simulink model "cordict1"  (R2023a)
settings: Solver=FixedStepAuto  StartTime=0.0  StopTime=60e-6  RelTol=1e-3
values from neighbouring files (symbols this model uses):
  FFTLength = 32    [matlab_channel.m]
  yr_c = yr_c(t,:)    [matlab_channel.m]
undefined symbols (not defined in the file or in its folder): Add, Shift
libraries: dspindex x4, dsphdlmathfun2 x1, dsphdlfiltering2 x1, dspsrcs4 x1
settings Model: Creator=Windows User  LastModifiedBy=Windows User
settings OptimizationCC: BlockReduction=off  ConditionallyExecuteInputs=off  DefaultParameterBehavior=Inlined
settings DebuggingCC: AlgebraicLoopMsg=error
settings HardwareCC: ProdBitPerPointer=32  ProdBitPerSizeT=32  ProdBitPerPtrDiffT=32  ProdLargestAtomicFloat=None  ProdIntDivRoundTo=Undefined  ProdEndianess=Unspecified  ProdWordSize=32  ProdHWDeviceType=ASIC/FPGA->ASIC/FPGA  TargetBitPerPointer=64  TargetBitPerSizeT=64  TargetBitPerPtrDiffT=64  TargetLongLongMode=on  TargetIntDivRoundTo=Zero  TargetEndianess=LittleEndian  TargetWordSize=64  TargetHWDeviceType=Custom Processor->MATLAB Host Computer  ProdEqTarget=off

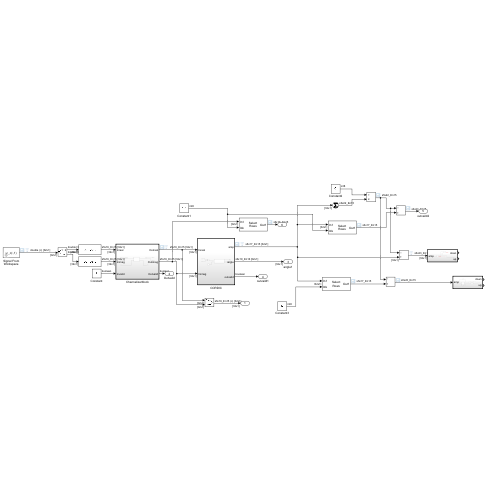
[thumbnail: Simulink's stored preview of the top-level diagram]
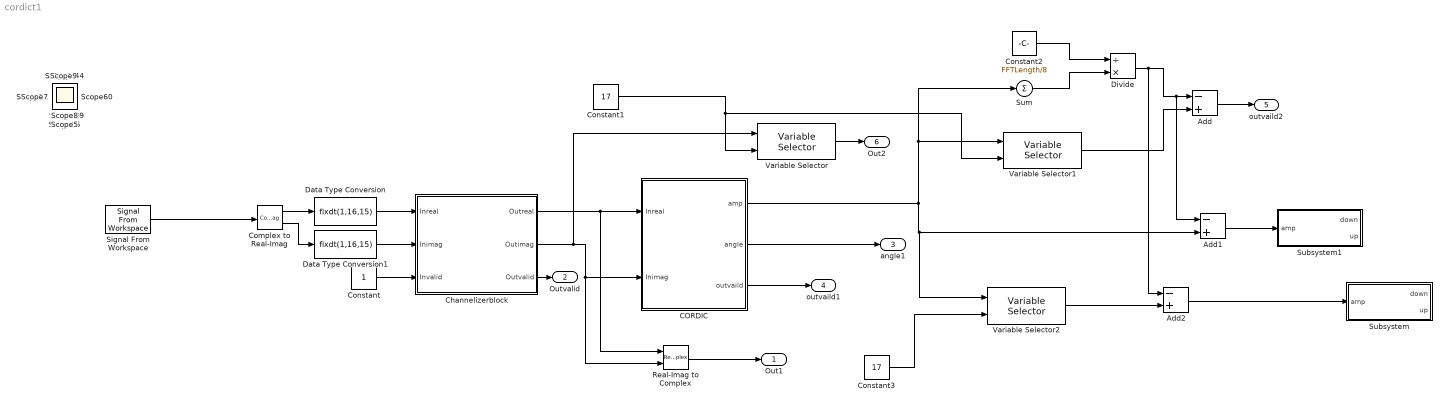
== system cordict1 ==
  Add : Sum  Inputs=-+
  Add1 : Sum  Inputs=-+
  Add2 : Sum  Inputs=-+
  CORDIC : Subsystem  TreatAsAtomicUnit=on
  Channelizerblock : Subsystem  TreatAsAtomicUnit=on
  Complex to Real-Imag : ComplexToRealImag
  Constant : Constant  VectorParams1D=off  OutDataTypeStr=boolean  SampleTime=-1
  Constant1 : Constant  Value=17  VectorParams1D=off  OutDataTypeStr=int8  SampleTime=-1
  Constant2 : Constant  Value=FFTLength/8  OutDataTypeStr=int8  SampleTime=-1
  Constant3 : Constant  Value=17  VectorParams1D=off  OutDataTypeStr=int8  SampleTime=-1
  Data Type Conversion : DataTypeConversion  OutDataTypeStr=fixdt(1,16,15)  SaturateOnIntegerOverflow=off  RndMeth=Floor  LockScale=on
  Data Type Conversion1 : DataTypeConversion  OutDataTypeStr=fixdt(1,16,15)  SaturateOnIntegerOverflow=off  RndMeth=Floor  LockScale=on
  Divide : Product  Inputs=/*
  Real-Imag to Complex : RealImagToComplex
  Signal From Workspace : dspsrcs4/Signal From Workspace  X=yr_c(:,1)  Ts=1/2e9  nsamps=FFTLength  OutputAfterFinalValue=Setting to zero  ignoreOrWarnInputAndFrameLengths=off  OutputFrames=off
  Subsystem : Subsystem  TreatAsAtomicUnit=on
  Subsystem1 : Subsystem  TreatAsAtomicUnit=on
  Sum : Sum  Inputs=+  CollapseMode=Specified dimension
  Variable Selector : dspindex/Variable Selector  NumInputs=1  rowsOrCols=Rows  IdxMode=Variable  Elements=[1 3]  ZerOneIdxMode=One-based  errmode=Clip Index  FillMode=off  FillValues=0
  Variable Selector1 : dspindex/Variable Selector  NumInputs=1  rowsOrCols=Rows  IdxMode=Variable  Elements=[1 3]  ZerOneIdxMode=One-based  errmode=Clip Index  FillMode=off  FillValues=0
  Variable Selector2 : dspindex/Variable Selector  NumInputs=1  rowsOrCols=Rows  IdxMode=Variable  Elements=[1 3]  ZerOneIdxMode=One-based  errmode=Clip Index  FillMode=off  FillValues=0
  Out1 : Outport  VectorParamsAs1DForOutWhenUnconnected=off
  Outvalid : Outport  Port=2  VectorParamsAs1DForOutWhenUnconnected=off
  angle1 : Outport  Port=3  VectorParamsAs1DForOutWhenUnconnected=off
  outvaild1 : Outport  Port=4  VectorParamsAs1DForOutWhenUnconnected=off
  outvaild2 : Outport  Port=5  VectorParamsAs1DForOutWhenUnconnected=off
  Out2 : Outport  Port=6
  Scope{,1..21} (22 alike) : Scope
  wires:
  Signal From Workspace/1 -> Complex to Real-Imag/1
  Data Type Conversion1/1 -> Channelizerblock/2(Inimag)
  Complex to Real-Imag/1 -> Data Type Conversion/1
  Complex to Real-Imag/2 -> Data Type Conversion1/1
  Constant1/1 -> Variable Selector/2, Variable Selector1/2
  Data Type Conversion/1 -> Channelizerblock/1(Inreal)
  Constant/1 -> Channelizerblock/3(Invalid)
  Channelizerblock/1(Outreal) -> Real-Imag to Complex/1, CORDIC/1(Inreal)
  Channelizerblock/2(Outimag) -> Variable Selector/1, Real-Imag to Complex/2, CORDIC/2(Inimag)
  Channelizerblock/3(Outvalid) -> Outvalid/1
  CORDIC/2(angle) -> angle1/1
  CORDIC/3(outvaild) -> outvaild1/1
  Real-Imag to Complex/1 -> Out1/1
  CORDIC/1(amp) -> Variable Selector2/1, Add1/2, Variable Selector1/1, Sum/1
  Sum/1 -> Divide/2
  Constant2/1 -> Divide/1
  Divide/1 -> Add2/1, Add1/1, Add/1
  Variable Selector1/1 -> Add/2
  Add/1 -> outvaild2/1
  Constant3/1 -> Variable Selector2/2
  Variable Selector2/1 -> Add2/2
  Add2/1 -> Subsystem/1(amp)
  Variable Selector/1 -> Out2/1
  Add1/1 -> Subsystem1/1(amp)

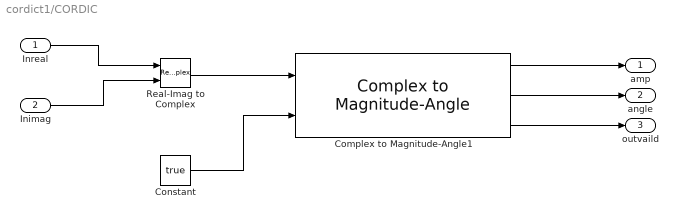
== system cordict1/CORDIC ==
  Inreal : Inport
  Inimag : Inport  Port=2
  Complex to Magnitude-Angle1 : dsphdlmathfun2/Complex to Magnitude-Angle  NumIterationsSource=Property  NumIterations=15  OutputFormat=Magnitude and angle  AngleFormat=Radians  ScaleOutput=on  ScalingMethod=Shift-Add  SimulateUsing=Code generation
  Constant : Constant  Value=true  OutDataTypeStr=boolean  LockScale=on
  Real-Imag to Complex : RealImagToComplex
  amp : Outport
  angle : Outport  Port=2
  outvaild : Outport  Port=3
  wires:
  Inimag/1 -> Real-Imag to Complex/2
  Real-Imag to Complex/1 -> Complex to Magnitude-Angle1/1
  Complex to Magnitude-Angle1/1 -> amp/1
  Constant/1 -> Complex to Magnitude-Angle1/2
  Complex to Magnitude-Angle1/3 -> outvaild/1
  Complex to Magnitude-Angle1/2 -> angle/1
  Inreal/1 -> Real-Imag to Complex/1

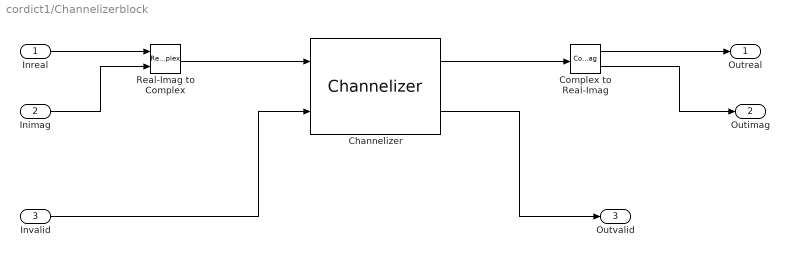
== system cordict1/Channelizerblock ==
  Inreal : Inport
  Inimag : Inport  Port=2
  Invalid : Inport  Port=3
  Channelizer : dsphdlfiltering2/Channelizer  FilterCoefficients=LowpassCoefficients  FilterStructure=Direct form transposed  NumFrequencyBands=FFTLength  ComplexMultiplication=Use 4 multipliers and 2 adders  Normalize=on  OutputSize=Same as input size  SimulateUsing=Code generation  roundingMode=Floor  overflowMode=off  CoefficientsDataTypeStr=Inherit: Same word length as input  FilterOutputDataTypeStr=fixdt(1,16,15)  ResetInputPort=off  StartOutputPort=off  EndOutputPort=off
  Complex to Real-Imag : ComplexToRealImag
  Real-Imag to Complex : RealImagToComplex
  Outreal : Outport
  Outimag : Outport  Port=2
  Outvalid : Outport  Port=3
  wires:
  Inreal/1 -> Real-Imag to Complex/1
  Inimag/1 -> Real-Imag to Complex/2
  Real-Imag to Complex/1 -> Channelizer/1
  Invalid/1 -> Channelizer/2
  Channelizer/1 -> Complex to Real-Imag/1
  Complex to Real-Imag/1 -> Outreal/1
  Complex to Real-Imag/2 -> Outimag/1
  Channelizer/2 -> Outvalid/1

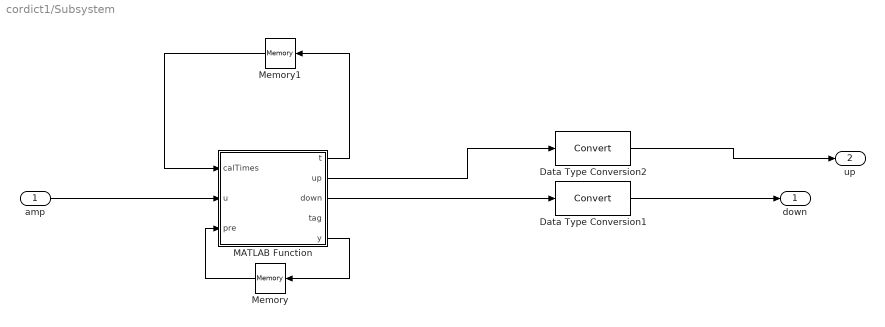
== system cordict1/Subsystem ==
  amp : Inport
  Data Type Conversion1 : DataTypeConversion  SaturateOnIntegerOverflow=off  RndMeth=Floor
  Data Type Conversion2 : DataTypeConversion  SaturateOnIntegerOverflow=off  RndMeth=Floor
  MATLAB Function : MATLAB Function  TreatAsAtomicUnit=on
  Memory : Memory  InheritSampleTime=on
  Memory1 : Memory  InheritSampleTime=on
  down : Outport
  up : Outport  Port=2
  wires:
  amp/1 -> MATLAB Function/2(u)
  MATLAB Function/5(y) -> Memory/1
  Memory/1 -> MATLAB Function/3(pre)
  MATLAB Function/1(t) -> Memory1/1
  Memory1/1 -> MATLAB Function/1(calTimes)
  MATLAB Function/3(down) -> Data Type Conversion1/1
  MATLAB Function/2(up) -> Data Type Conversion2/1
  Data Type Conversion2/1 -> up/1
  Data Type Conversion1/1 -> down/1

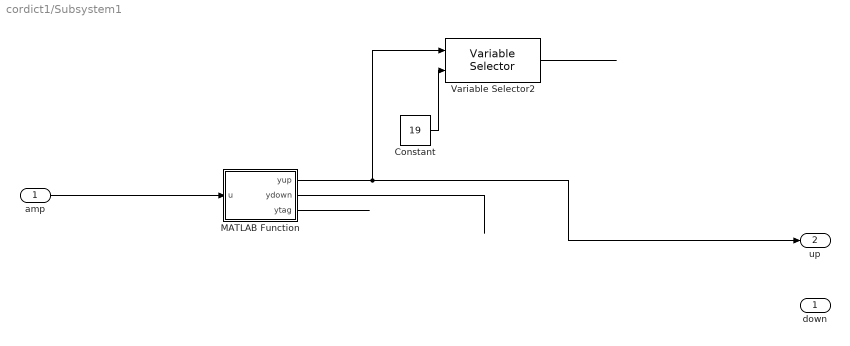
== system cordict1/Subsystem1 ==
  amp : Inport
  Constant : Constant  Value=19  SampleTime=-1
  MATLAB Function : MATLAB Function  TreatAsAtomicUnit=on
  Variable Selector2 : dspindex/Variable Selector  NumInputs=1  rowsOrCols=Rows  IdxMode=Variable  Elements=[1 3]  ZerOneIdxMode=One-based  errmode=Clip Index  FillMode=off  FillValues=0
  down : Outport
  up : Outport  Port=2
  wires:
  amp/1 -> MATLAB Function/1(u)
  MATLAB Function/1(yup) -> Variable Selector2/1, up/1
  MATLAB Function/2(ydown) -> ?
  MATLAB Function/3(ytag) -> ?
  Constant/1 -> Variable Selector2/2
  Variable Selector2/1 -> ?

== matlab function cordict1/Subsystem1/MATLAB Function ==
  data: u input; yup output; ydown output; ytag output
function [yup, ydown, ytag]= fcn(u)
    persistent time;
    persistent up;
    persistent up_times;
    persistent down;
    persistent tag;
    if isempty(time)
        time = 0;
        up = zeros(32,1);
        up_times = zeros(32,1);
        down = zeros(32,1);
        tag = zeros(32,1);
    end
    for i = 1:32
        if u(i) >= 0
            up_times(i) = up_times(i) + 1;
            if up_times(i) >= 50 && up(i) == 0
                up(i) = time;
                tag(i) = 1;
            end
        else
            up_times(i) = 0;
            if up(i) ~= 0
                down(i) = time;
            end
        end
    end

    time = time + 1;
    yup = up;
    ydown = down;
    ytag = tag;

== matlab function cordict1/Subsystem/MATLAB Function ==
  data: calTimes input; t output; up output; down output; tag output; u input; y output; pre input
function [t, up, down, tag, y] = fcn(calTimes, u, pre)
up = 0 ;
down = 0;
tag = 0;
t = calTimes + 1;
%#codegen
if u>0
    y = pre + 1;
else 
    y = 0;
end


if pre == 18 && y > 18
    up = calTimes;
    tag = 1;
end

if pre>18 && y == 0
    down = t;
end
